simulink model "DynamicModel_pro"  (R2022a)
settings: Solver=ode4  StartTime=0.0  StopTime=10  FixedStep=0.1  MaxStep=1e-5  RelTol=1e-10
InitFcn:
  | SM_Data
StopFcn:
  | forPlot
values from neighbouring files (symbols this model uses):
  d_Phi_b = [0,0,0].'    [SM_Data.m]
  d_theta_m = [0,0,0,0].'    [SM_Data.m]
  H_b = [1.2,0,-0.3;1,0.89,0.24;0.36,0,0.21]    [SM_Data.m]
  Kdbf = diag([5,4,4],0)    [SM_Data.m]
  Kdmf = diag([2,2.3,2.5,2.5],0)    [SM_Data.m]
  Kibc = diag([0.9,0.96,1.2],0)    [SM_Data.m]
  Kimc = diag([0.9,0.89,0.98,0.9],0)    [SM_Data.m]
  Kpbc = diag([5.33,4.2,5.1],0)    [SM_Data.m]
  Kpbf = diag([5,5.1,5.2],0)    [SM_Data.m]
  Kpmc = diag([5.1,5.5,5.1,5.4],0)    [SM_Data.m]
  Kpmf = diag([4,3,2,2],0)    [SM_Data.m]
  Phi_b = [0.8,-0.6,0.5].'    [SM_Data.m]
  Phi_b_d = [0.2,0.1,0.3].'    [SM_Data.m]
  theta_m = [1.5,0.7,1.0,2.3].'    [SM_Data.m]
  theta_m_d = [0.3,0.4,0.5,0.6].'    [SM_Data.m]
settings Model: Creator=Zou Xiangxiang  LastModifiedBy=43840
settings SolverCC: ZeroCrossAlgorithm=Adaptive

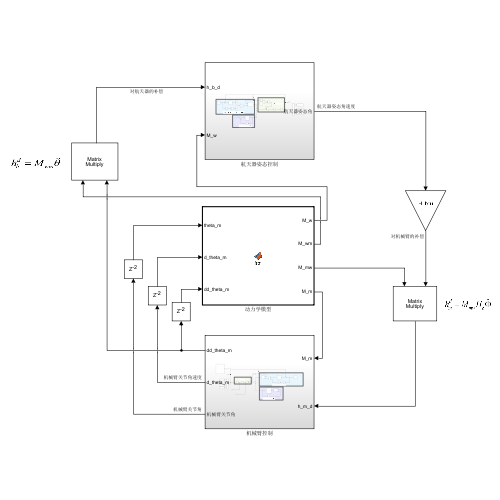
[thumbnail: Simulink's stored preview of the top-level diagram]
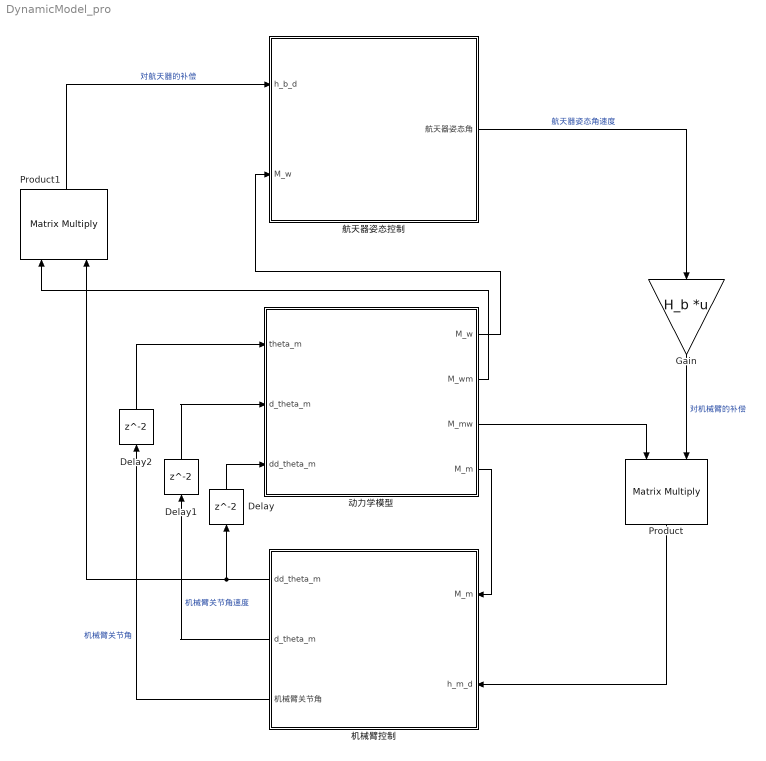
== system DynamicModel_pro ==
  Delay : Delay
  Delay1 : Delay
  Delay2 : Delay
  Gain : Gain  Gain=H_b  Multiplication=Matrix(K*u)
  Product : Product  Multiplication=Matrix(*)
  Product1 : Product  Multiplication=Matrix(*)
  动力学模型 : MATLAB Function  TreatAsAtomicUnit=on
  机械臂控制 : Subsystem
  航天器姿态控制 : Subsystem
  wires:
  航天器姿态控制/1(航天器姿态角) -> Gain/1  "航天器姿态角速度"
  Product1/1 -> 航天器姿态控制/1(h_b_d)  "对航天器的补偿"
  机械臂控制/2(d_theta_m) -> Delay1/1  "机械臂关节角速度"
  机械臂控制/3(机械臂关节角) -> Delay2/1  "机械臂关节角"
  Gain/1 -> Product/2  "对机械臂的补偿"
  Product/1 -> 机械臂控制/2(h_m_d)
  机械臂控制/1(dd_theta_m) -> Delay/1, Product1/2
  动力学模型/2(M_wm) -> Product1/1
  动力学模型/3(M_mw) -> Product/1
  动力学模型/4(M_m) -> 机械臂控制/1(M_m)
  动力学模型/1(M_w) -> 航天器姿态控制/2(M_w)
  Delay/1 -> 动力学模型/3(dd_theta_m)
  Delay1/1 -> 动力学模型/2(d_theta_m)
  Delay2/1 -> 动力学模型/1(theta_m)

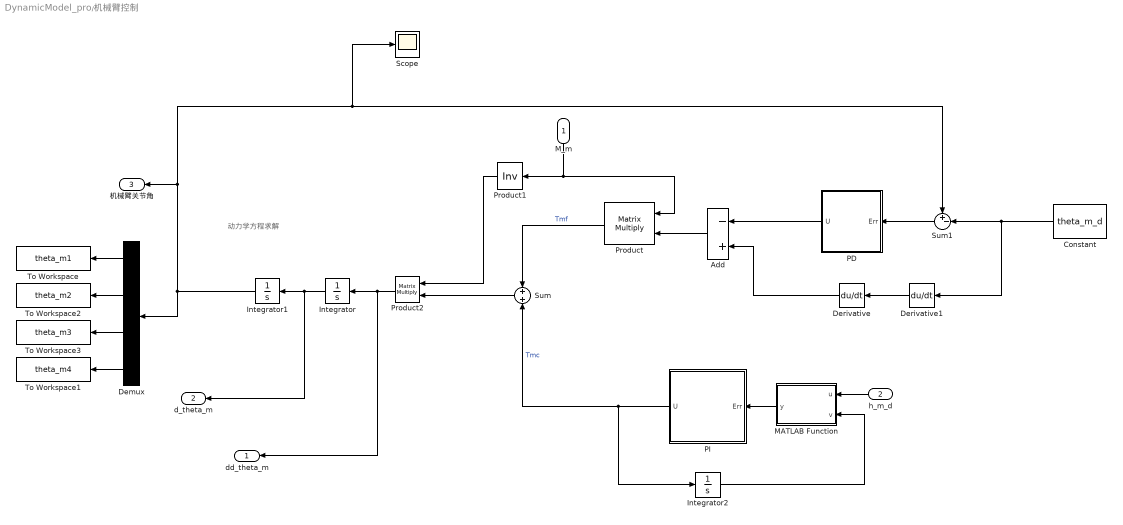
== system DynamicModel_pro/机械臂控制 ==
  note: 动力学方程求解
  M_m : Inport
  h_m_d : Inport  Port=2
  Add : Sum  Inputs=-+
  Constant : Constant  Value=theta_m_d
  Demux : Demux
  Derivative : Derivative
  Derivative1 : Derivative
  Integrator : Integrator  InitialCondition=d_theta_m  UpperSaturationLimit=2  LowerSaturationLimit=-2
  Integrator1 : Integrator  InitialCondition=theta_m  UpperSaturationLimit=5  LowerSaturationLimit=-5
  Integrator2 : Integrator
  MATLAB Function : MATLAB Function  TreatAsAtomicUnit=on
  PD : Subsystem
  PI : Subsystem
  Product : Product  Multiplication=Matrix(*)
  Product1 : Product  Inputs=/  Multiplication=Matrix(*)
  Product2 : Product  Multiplication=Matrix(*)
  Scope : Scope
  Sum : Sum  Inputs=+|+
  Sum1 : Sum  Inputs=+-|
  To Workspace : ToWorkspace  VariableName=theta_m1  SampleTime=-1
      settings: Save2DSignal=2-D array (concatenate along first dimension)
  To Workspace1 : ToWorkspace  VariableName=theta_m4  SampleTime=-1
      settings: Save2DSignal=2-D array (concatenate along first dimension)
  To Workspace2 : ToWorkspace  VariableName=theta_m2  SampleTime=-1
      settings: Save2DSignal=2-D array (concatenate along first dimension)
  To Workspace3 : ToWorkspace  VariableName=theta_m3  SampleTime=-1
      settings: Save2DSignal=2-D array (concatenate along first dimension)
  dd_theta_m : Outport
  d_theta_m : Outport  Port=2
  机械臂关节角 : Outport  Port=3
  wires:
  Integrator2/1 -> MATLAB Function/2(v)
  Integrator/1 -> Integrator1/1, d_theta_m/1
  PI/1(U) -> Sum/2, Integrator2/1  "Tmc"
  MATLAB Function/1(y) -> PI/1(Err)
  Integrator1/1 -> Demux/1, Scope/1, Sum1/1, 机械臂关节角/1
  Product2/1 -> Integrator/1, dd_theta_m/1
  Derivative1/1 -> Derivative/1
  Sum1/1 -> PD/1(Err)
  Product/1 -> Sum/1  "Tmf"
  Add/1 -> Product/2
  PD/1(U) -> Add/1
  Derivative/1 -> Add/2
  h_m_d/1 -> MATLAB Function/1(u)
  M_m/1 -> Product1/1, Product/1
  Sum/1 -> Product2/2
  Product1/1 -> Product2/1
  Demux/1 -> To Workspace/1
  Demux/2 -> To Workspace2/1
  Demux/3 -> To Workspace3/1
  Demux/4 -> To Workspace1/1
  Constant/1 -> Derivative1/1, Sum1/2

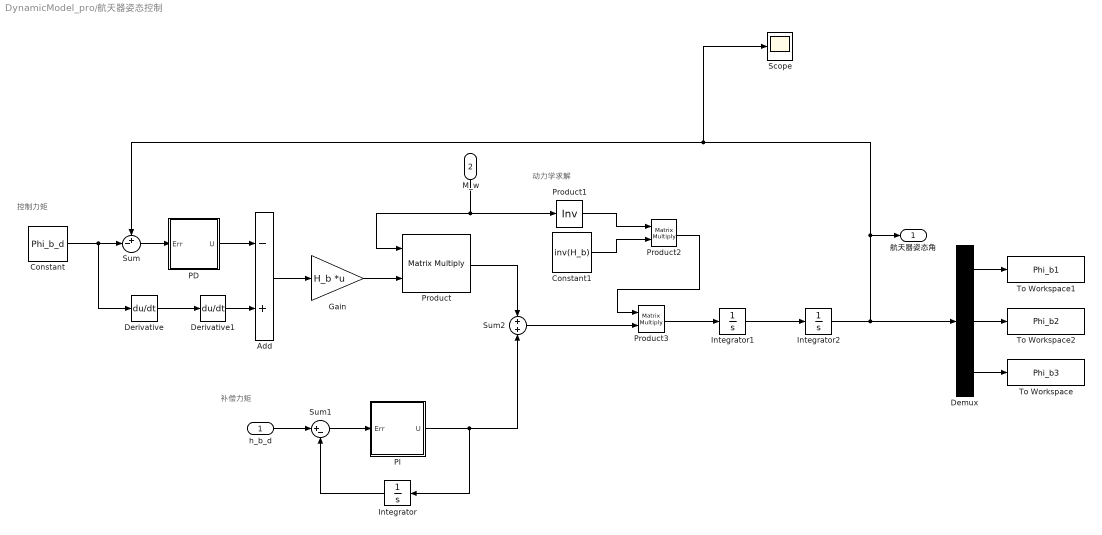
== system DynamicModel_pro/航天器姿态控制 ==
  note: 动力学求解
  note: 补偿力矩
  note: 控制力矩
  h_b_d : Inport
  M_w : Inport  Port=2
  Add : Sum  Inputs=-+
  Constant : Constant  Value=Phi_b_d  VectorParams1D=off
  Constant1 : Constant  Value=inv(H_b)
  Demux : Demux  Outputs=3
  Derivative : Derivative
  Derivative1 : Derivative
  Gain : Gain  Gain=H_b  Multiplication=Matrix(K*u)
  Integrator : Integrator
  Integrator1 : Integrator  InitialCondition=d_Phi_b
  Integrator2 : Integrator  InitialCondition=Phi_b
  PD : Subsystem
  PI : Subsystem
  Product : Product  Multiplication=Matrix(*)
  Product1 : Product  Inputs=/  Multiplication=Matrix(*)
  Product2 : Product  Multiplication=Matrix(*)
  Product3 : Product  Multiplication=Matrix(*)
  Scope : Scope
  Sum : Sum  Inputs=+-|
  Sum1 : Sum  Inputs=|+-
  Sum2 : Sum  Inputs=+|+
  To Workspace : ToWorkspace  VariableName=Phi_b3  SampleTime=-1
      settings: Save2DSignal=2-D array (concatenate along first dimension)
  To Workspace1 : ToWorkspace  VariableName=Phi_b1  SampleTime=-1
      settings: Save2DSignal=2-D array (concatenate along first dimension)
  To Workspace2 : ToWorkspace  VariableName=Phi_b2  SampleTime=-1
      settings: Save2DSignal=2-D array (concatenate along first dimension)
  航天器姿态角 : Outport
  wires:
  Sum/1 -> PD/1(Err)
  Integrator/1 -> Sum1/2
  Product3/1 -> Integrator1/1
  Sum1/1 -> PI/1(Err)
  Derivative/1 -> Derivative1/1
  PD/1(U) -> Add/1
  Add/1 -> Gain/1
  Sum2/1 -> Product3/2
  PI/1(U) -> Sum2/2, Integrator/1
  h_b_d/1 -> Sum1/1
  Integrator1/1 -> Integrator2/1
  Derivative1/1 -> Add/2
  Constant/1 -> Derivative/1, Sum/2
  M_w/1 -> Product/1, Product1/1
  Gain/1 -> Product/2
  Product/1 -> Sum2/1
  Product1/1 -> Product2/1
  Constant1/1 -> Product2/2
  Product2/1 -> Product3/1
  Integrator2/1 -> Demux/1, Scope/1, Sum/1, 航天器姿态角/1
  Demux/1 -> To Workspace1/1
  Demux/2 -> To Workspace2/1
  Demux/3 -> To Workspace/1

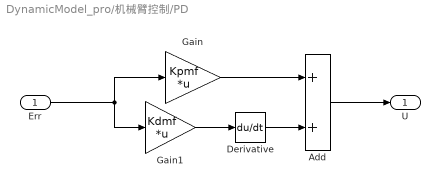
== system DynamicModel_pro/机械臂控制/PD ==
  Err : Inport
  Add : Sum
  Derivative : Derivative
  Gain : Gain  Gain=Kpmf  Multiplication=Matrix(K*u)
  Gain1 : Gain  Gain=Kdmf  Multiplication=Matrix(K*u)
  U : Outport
  wires:
  Err/1 -> Gain1/1, Gain/1
  Gain1/1 -> Derivative/1
  Gain/1 -> Add/1
  Derivative/1 -> Add/2
  Add/1 -> U/1

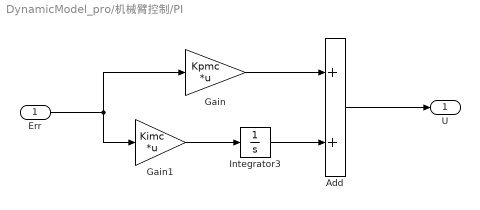
== system DynamicModel_pro/机械臂控制/PI ==
  Err : Inport
  Add : Sum
  Gain : Gain  Gain=Kpmc  Multiplication=Matrix(K*u)
  Gain1 : Gain  Gain=Kimc  Multiplication=Matrix(K*u)
  Integrator3 : Integrator
  U : Outport
  wires:
  Gain1/1 -> Integrator3/1
  Add/1 -> U/1
  Gain/1 -> Add/1
  Err/1 -> Gain1/1, Gain/1
  Integrator3/1 -> Add/2

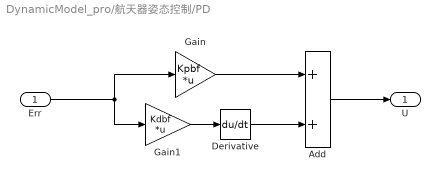
== system DynamicModel_pro/航天器姿态控制/PD ==
  Err : Inport
  Add : Sum
  Derivative : Derivative
  Gain : Gain  Gain=Kpbf  Multiplication=Matrix(K*u)
  Gain1 : Gain  Gain=Kdbf  Multiplication=Matrix(K*u)
  U : Outport
  wires:
  Err/1 -> Gain1/1, Gain/1
  Gain1/1 -> Derivative/1
  Gain/1 -> Add/1
  Derivative/1 -> Add/2
  Add/1 -> U/1

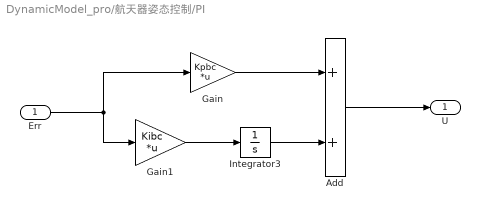
== system DynamicModel_pro/航天器姿态控制/PI ==
  Err : Inport
  Add : Sum
  Gain : Gain  Gain=Kpbc  Multiplication=Matrix(K*u)
  Gain1 : Gain  Gain=Kibc  Multiplication=Matrix(K*u)
  Integrator3 : Integrator
  U : Outport
  wires:
  Gain1/1 -> Integrator3/1
  Add/1 -> U/1
  Gain/1 -> Add/1
  Err/1 -> Gain1/1, Gain/1
  Integrator3/1 -> Add/2

== matlab function DynamicModel_pro/机械臂控制/MATLAB Function ==
  data: u input; y output; v input
function y = fcn(u,v)

y = u-v;

== matlab function DynamicModel_pro/动力学模型 ==
  data: theta_m input; M_w output; M_wm output; M_mw output; M_m output; d_theta_m input; dd_theta_m input
function [M_w, M_wm, M_mw, M_m] = fcn(theta_m, d_theta_m, dd_theta_m)
%% 连接外部m文件
coder.extrinsic("Mass")     

%% 初始化
M_w=zeros(3,3);
M_wm=zeros(3,4);
M_mw=zeros(4,3);
M_m=zeros(4,4);

%% 返回质量矩阵
[M_w, M_wm, M_mw, M_m]=Mass(theta_m, d_theta_m, dd_theta_m);
